simulink model "hmi_view_manager_02"  (Simulink 7.0)
settings: Solver=ode45  StartTime=0.0  StopTime=inf  RelTol=1e-3
settings Model: Creator=emanoj1  LastModifiedBy=ARAJASE2

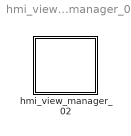
== system hmi_view_manager_02 ==
  hmi_view_manager_02 : Stateflow chart

== stateflow chart hmi_view_manager_02 ==
  settings: executeAtInitialization=1
  state VM_LOGIC_ST [parallel]
    /*
    ** Maintains the request from HMI logic
    */
    settings: executionOrder=1
    state VM_LOGIC_ACTIVE_ST
      entry:
      l_logic_active_state_id = p_logic_req_state_id;
      l_logic_active_anim_id = p_logic_req_anim_id;
      exit:
      l_logic_active_state_id = LSH_ALL_VM_LOGIC_STATES;
      l_logic_active_anim_id = ANIM_MAX_ID;
      VM_LOGIC_ACTIVE_ST -> (junction 29) [order 1] : LSH_LOGIC_ADD_EV
          | [p_logic_req_state_id < LSH_ALL_VM_LOGIC_STATES]
      (junction 29) -> (junction 30) [order 1] : /* New state is replacing current state */
          | [l_logic_active_state_id != p_logic_req_state_id]
      (junction 61) -> (junction 34)
      (junction 29) -> (junction 32) [order 2] : /* requested state is same as active state */
      (junction 30) -> (junction 33) [order 1] : [(p_logic_req_state_id == l_gfx_active_state_id) &&...
          | (!in(VM_GFX_CLOSE_ANIM_ST))]
          | {l_gfx_deactivate_flag = FALSE;}
      (junction 31) -> (junction 34) [order 2] : /*
          | ** active state is not being presented yet by graphics
          | ** so no deactivations required
          | */
      (junction 32) -> (junction 33) [order 2] : /* req state prev anim actively running */
      (junction 34) -> (junction 33)
      (junction 33) -> VM_LOGIC_ACTIVE_ST : {
          |    l_logic_active_state_id = p_logic_req_state_id;
          |    l_logic_active_anim_id = p_logic_req_anim_id;
          | }
      (junction 32) -> (junction 64) [order 1] : [(l_gfx_active_anim_id == ANIM_MAX_ID) ]
          | {
          | $#ifdef LSH_IGNORE_ANIM_REQUEST_DURING_ACTIVE_ANIM$
          |    l_logic_active_anim_id = ANIM_MAX_ID;
          | $#else$
          |    l_logic_active_anim_id = p_logic_req_anim_id;
          | $#endif$
          | }
      (junction 30) -> (junction 31) [order 2]
      (junction 31) -> (junction 60) [order 1] : /*
          | ** active state is being presented by graphics so
          | ** need to deactivate it
          | */
          | [l_logic_active_state_id == l_gfx_active_state_id]
          | {l_gfx_deactivate_flag = TRUE;
          |  l_gfx_deactivate_anim = ANIM_MAX_ID;}
      (junction 60) -> (junction 61)
      (junction 64) -> VM_LOGIC_ACTIVE_ST [order 2]
      (junction 64) -> (junction 62) [order 1] : [l_logic_active_anim_id ==ANIM_ABORT_ID]
      (junction 62) -> VM_LOGIC_ACTIVE_ST : {
          |  l_logic_active_anim_id = ANIM_MAX_ID;
          | }
    state VM_LOGIC_INACTIVE_ST
      (junction 73) -> VM_LOGIC_INACTIVE_ST [order 1] : [ (p_logic_req_anim_id==ANIM_ABORT_ID)]
          | {l_gfx_deactivate_anim = p_logic_req_anim_id;}
      VM_LOGIC_INACTIVE_ST -> (junction 68) [order 1] : LSH_LOGIC_REMOVE_EV
          | [(p_logic_req_state_id == l_gfx_active_state_id) ]
      (junction 68) -> (junction 69) [order 1] : [! in(VM_GFX_CLOSE_ANIM_ST)]
      (junction 69) -> VM_LOGIC_INACTIVE_ST : {l_gfx_deactivate_anim = p_logic_req_anim_id;}
      (junction 68) -> (junction 73) [order 2]
      (junction 73) -> (junction 74) [order 2]
      (junction 74) -> VM_LOGIC_INACTIVE_ST : /* Do Nothing*/
          | /* QAC 8.1.2 Fix*/
    (default) -> VM_LOGIC_INACTIVE_ST
    VM_LOGIC_INACTIVE_ST -> (junction 25) [order 1] : LSH_LOGIC_ADD_EV
        | [p_logic_req_state_id < LSH_ALL_VM_LOGIC_STATES]
    (junction 25) -> VM_LOGIC_ACTIVE_ST
    (junction 27) -> VM_LOGIC_INACTIVE_ST [order 1] : [p_logic_req_state_id == l_gfx_active_state_id]
        | {l_gfx_deactivate_flag = TRUE;
        |  l_gfx_deactivate_anim = p_logic_req_anim_id;}
    VM_LOGIC_ACTIVE_ST -> (junction 27) [order 1] : LSH_LOGIC_REMOVE_EV
        | [p_logic_req_state_id == l_logic_active_state_id]
    (junction 27) -> (junction 28) [order 2]
    (junction 28) -> VM_LOGIC_INACTIVE_ST
  state VM_PRESENTATION_ST [parallel]
    /*
    ** Maintains the graphics state
    */
    settings: executionOrder=2
    state VM_GFX_ACTIVE_ST
      entry:
      l_gfx_prev_focus = 0;
      l_gfx_deactivate_flag = FALSE;
      state VM_GFX_NORMAL_RUN_ST
        state VM_GFX_ACTIVE_PRESENT_ST
          entry:
          l_logic_active_anim_id = ANIM_MAX_ID; /*Added during Abort anim implementation */
          hmi_vm_focus(l_gfx_active_state_id, ...
          (LSH_GOT_FOCUS_STATUS|LSH_ANIM_COMPLETE_STATUS));
          hmi_lsh_run_presentation(l_gfx_active_state_id,l_gfx_presentation_state);
          l_gfx_presentation_state = LSH_REFRESH_STATUS;
          /*Added during Abort anim implementation */
          l_gfx_active_anim_id = ANIM_MAX_ID;
          VM_GFX_ACTIVE_PRESENT_ST -> (junction 65) : /* call refresh every alternate cycles */
              | LSH_GFX_TICK_EV
              | {hmi_lsh_run_presentation(l_gfx_active_state_id, LSH_REFRESH_STATUS);}
          (junction 65) -> VM_GFX_ACTIVE_PRESENT_ST [order 1] : [l_logic_active_anim_id==ANIM_ABORT_ID]
              | {l_logic_active_anim_id = ANIM_MAX_ID;}
          (junction 66) -> VM_GFX_ACTIVE_PRESENT_ST
          (junction 65) -> (junction 66) [order 2]
        state VM_GFX_ACTIVE_ANIMATION_ST
          entry:
          hmi_vm_focus(l_gfx_active_state_id,(LSH_GOT_FOCUS_STATUS|LSH_ANIM_STARTED_STATUS));
          on LSH_GFX_FORCE_PRESENTATION_EV:
          hmi_lsh_run_presentation(l_gfx_active_state_id,l_gfx_presentation_state);
          l_gfx_presentation_state = LSH_REFRESH_STATUS;
        (junction 48) -> (junction 41) [order 1] : [l_logic_active_anim_id < ANIM_MAX_ID]
        (default) -> (junction 48)
        (junction 41) -> (junction 40) : {
            |    hmi_lsh_stop_animation(l_gfx_active_state_id, l_gfx_active_anim_id);
            |    l_gfx_active_anim_id     = l_logic_active_anim_id;
            |    l_logic_active_anim_id  = ANIM_MAX_ID;
            | }
        (junction 40) -> VM_GFX_ACTIVE_ANIMATION_ST [order 1] : /*
            | ** !!!!! This transition needs to be avaluated first always
            | ** So if for any chance if you rearrange the states
            | ** please make sure the order is maintained
            | */
            | [hmi_lsh_start_animation(l_gfx_active_state_id, l_gfx_active_anim_id) != FALSE]
        (junction 63) -> (junction 41)
        VM_GFX_NORMAL_RUN_ST -> (junction 63) : LSH_GFX_TICK_EV
            | [l_logic_active_anim_id < ANIM_MAX_ID]
            | /* if logic active state is different, it will exit
            | in parent state  */
        (junction 47) -> VM_GFX_ACTIVE_PRESENT_ST : [!in(VM_GFX_ACTIVE_PRESENT_ST)]
        VM_GFX_ACTIVE_ANIMATION_ST -> (junction 63) [order 1] : LSH_ANIM_COMPLETE_EV
        (junction 40) -> (junction 47) [order 2]
        (junction 48) -> VM_GFX_ACTIVE_PRESENT_ST [order 2]
        (junction 42) -> (junction 47) : LSH_GFX_TICK_EV
            | [(l_logic_active_anim_id==ANIM_ABORT_ID)&&...
            |         (l_gfx_active_state_id==l_logic_active_state_id)]
            | {
            | hmi_lsh_stop_animation(l_gfx_active_state_id, l_gfx_active_anim_id);
            | l_logic_active_anim_id=ANIM_MAX_ID;
            | }
        VM_GFX_ACTIVE_ANIMATION_ST -> (junction 42) [order 2]
      state VM_GFX_STARTUP_ANIM_ST
        entry:
        hmi_vm_focus(l_gfx_active_state_id, (LSH_GOT_FOCUS_STATUS|LSH_ANIM_STARTED_STATUS));
        on LSH_GFX_FORCE_PRESENTATION_EV:
        hmi_lsh_run_presentation(l_gfx_active_state_id,l_gfx_presentation_state);
        l_gfx_presentation_state = LSH_REFRESH_STATUS;
      note: When entering for the first time see if we need to run a startup anim
          | While doing startup anim, if there is a request to run presentaion do it.
          | Once the startup anim is complete, enter normal  mode and do
          | presentation
          | In normal mode if the animation is requested perform that
      (default) -> (junction 43)
      (junction 35) -> VM_GFX_NORMAL_RUN_ST [order 1] : /* no animations */
          | [hmi_lsh_start_animation(l_gfx_active_state_id, l_gfx_active_anim_id)==FALSE]
      (junction 35) -> (junction 36) [order 2]
      VM_GFX_STARTUP_ANIM_ST -> VM_GFX_NORMAL_RUN_ST [order 2] : LSH_ANIM_COMPLETE_EV
      (junction 36) -> VM_GFX_STARTUP_ANIM_ST
      VM_GFX_ACTIVE_ST -> (junction 43) [order 1] : LSH_GFX_TICK_EV
          | [(l_gfx_active_state_id != l_logic_active_state_id)]
          | {
          |    l_gfx_prev_focus = 0;
          |    hmi_lsh_run_presentation(l_gfx_active_state_id, ...
          |                                        LSH_DEACTIVATED_STATUS);
          |    hmi_vm_focus(l_gfx_active_state_id, ...
          |                                (LSH_LOST_FOCUS_STATUS|...
          |                                 LSH_DEACTIVATED_STATUS|...
          |                                 LSH_ANIM_COMPLETE_STATUS));
          |    hmi_lsh_freeze_button_events_ext(LSH_GET_STATE_ID(l_gfx_active_state_id), ...
          |                                                                     LSH_GET_CLIENT_ID(l_gfx_active_state_id));
          | }
          | /*
          | Force a reentry if the logic state is different than
          | the current graphics state
          | This path is never expected to execute
          | */
      (junction 43) -> (junction 35) : {
          |    hmi_lsh_stop_animation(l_gfx_active_state_id, l_gfx_active_anim_id);
          |    l_gfx_active_state_id       = l_logic_active_state_id;
          |    l_gfx_active_anim_id       = l_logic_active_anim_id;
          |    l_logic_active_anim_id    = ANIM_MAX_ID;
          |    l_gfx_presentation_state = LSH_ACTIVATED_STATUS;
          | }
      VM_GFX_STARTUP_ANIM_ST -> VM_GFX_NORMAL_RUN_ST [order 1] : LSH_GFX_TICK_EV
          | [(l_logic_active_anim_id==ANIM_ABORT_ID)&&...
          |         (l_gfx_active_state_id==l_logic_active_state_id)]
          | {
          | hmi_lsh_stop_animation(l_gfx_active_state_id, l_gfx_active_anim_id);
          | l_logic_active_anim_id=ANIM_MAX_ID;
          | }
    state VM_GFX_INACTIVE_ST
      entry:
      l_gfx_active_state_id     = LSH_ALL_VM_LOGIC_STATES;
      l_gfx_active_anim_id     = ANIM_MAX_ID;
    state VM_GFX_CLOSE_ANIM_ST
      entry:
      l_gfx_active_anim_id = l_gfx_deactivate_anim;
      l_gfx_deactivate_anim = ANIM_MAX_ID;
    (default) -> VM_GFX_INACTIVE_ST
    VM_GFX_INACTIVE_ST -> VM_GFX_ACTIVE_ST : /* Check if we have got a new logic state */
        | LSH_GFX_TICK_EV
        | [l_logic_active_state_id < LSH_ALL_VM_LOGIC_STATES]
    VM_GFX_ACTIVE_ST -> (junction 37) [order 1] : /*
        | ** If the logic state has gone inactive or if the deactivation flag is set
        | ** then perform a deactivation. Perform the animation if requested
        | */
        | LSH_GFX_TICK_EV||...
        | LSH_GFX_CHECK_DEACTIVATION_EV||...
        | LSH_ANIM_COMPLETE_EV
        | [(l_logic_active_state_id == LSH_ALL_VM_LOGIC_STATES) || ...
        |  (l_gfx_deactivate_flag != FALSE)]
        | {
        |     hmi_lsh_stop_animation(l_gfx_active_state_id, l_gfx_active_anim_id);
        | }
    (junction 37) -> VM_GFX_CLOSE_ANIM_ST [order 1] : [hmi_lsh_start_animation(l_gfx_active_state_id, l_gfx_deactivate_anim) != FALSE]
    (junction 37) -> (junction 72) [order 2] : /* Animation not started */
    (junction 38) -> (junction 44) [order 2]
    VM_GFX_CLOSE_ANIM_ST -> (junction 39) [order 2] : /* animation completed and no state active */
        | LSH_ANIM_COMPLETE_EV
    (junction 39) -> (junction 72)
    (junction 44) -> VM_GFX_INACTIVE_ST [order 2]
    (junction 44) -> VM_GFX_ACTIVE_ST [order 1] : /* if we come here via l_gfx_deactivate_flag != FALSE path
        |    then check to see if there is an active state beccause
        |   focus handler can add/remove states */
        | [l_logic_active_state_id < LSH_ALL_VM_LOGIC_STATES]
    (junction 67) -> (junction 39)
    VM_GFX_CLOSE_ANIM_ST -> (junction 67) [order 1] : LSH_GFX_TICK_EV
        | [l_gfx_deactivate_anim==ANIM_ABORT_ID]
        | {
        |      hmi_lsh_stop_animation(l_gfx_active_state_id, l_gfx_active_anim_id);
        |     l_gfx_deactivate_anim=ANIM_MAX_ID;
        | }
    (junction 38) -> (junction 71) [order 1] : [(l_gfx_active_state_id != l_logic_active_state_id)]
    (junction 71) -> (junction 70) : {
        | hmi_lsh_freeze_button_events_ext(LSH_GET_STATE_ID(l_gfx_active_state_id), ...
        |                                                  LSH_GET_CLIENT_ID(l_gfx_active_state_id));
        | }
    (junction 70) -> (junction 44)
    (junction 72) -> (junction 38) : {
        | hmi_lsh_run_presentation(l_gfx_active_state_id,LSH_DEACTIVATED_STATUS);
        |    hmi_vm_focus(l_gfx_active_state_id, ...
        |                              (LSH_LOST_FOCUS_STATUS|...
        |                               LSH_DEACTIVATED_STATUS|...
        |                               LSH_ANIM_COMPLETE_STATUS));
        | }
  state hmi_vm_focus(p_state_id, p_focus) [function]
    (junction 54) -> (junction 26) : {
        |    hmi_lsh_focus_handler(p_state_id, p_focus);
        |    l_gfx_prev_focus = p_focus;
        | }
    (default) -> (junction 54)
  state hmi_vm_tick [function]
    (default) -> (junction 45) : {
        |    send(LSH_GFX_TICK_EV, VM_PRESENTATION_ST);
        |    send(LSH_GFX_TICK_EV, VM_PERIODIC_FOCUS_MONITOR_ST);
        | }
  state hmi_vm_check_deactivation [function]
    (default) -> (junction 50) : {
        |    send(LSH_GFX_CHECK_DEACTIVATION_EV, VM_PRESENTATION_ST);
        | }
  state hmi_vm_animation_completed [function]
    (default) -> (junction 53) : {
        |    send(LSH_ANIM_COMPLETE_EV, VM_PRESENTATION_ST);
        | }
  state hmi_vm_force_presentation [function]
    (default) -> (junction 46) : {
        |    send(LSH_GFX_FORCE_PRESENTATION_EV, VM_PRESENTATION_ST);
        | }
  state VM_PERIODIC_FOCUS_MONITOR_ST [parallel]
    settings: executionOrder=3
    note: This state will periodically invoke the focus handler to make sure that if a higher priority state got deactivated
        | then if this is the active state, appropriately set the got focus notification. Because the deactivated high
        | priority state will not initiate a got focus notification for next low priority state. It is this peridic check that
        | detects and generates the notification in such case
    VM_PERIODIC_FOCUS_MONITOR_ST -> (junction 49) : LSH_GFX_TICK_EV
        | [!in(VM_GFX_INACTIVE_ST)]
    (junction 49) -> VM_PERIODIC_FOCUS_MONITOR_ST : [hmi_lsh_get_focus_status(LSH_GET_STATE_ID(l_gfx_active_state_id)) == LSH_FOCUS_STATUS_INACTIVE]
        | {hmi_vm_focus(l_gfx_active_state_id, l_gfx_prev_focus);}
  state hmi_vm_add_state(p_state_id, p_anim_id) [function]
    (default) -> (junction 51) : {
        |    p_logic_req_state_id = p_state_id;
        |    p_logic_req_anim_id = p_anim_id;
        |    send(LSH_LOGIC_ADD_EV, VM_LOGIC_ST);
        | }
  state hmi_vm_remove_state(p_state_id, p_anim_id) [function]
    (default) -> (junction 52) : {
        |    p_logic_req_state_id = p_state_id;
        |    p_logic_req_anim_id = p_anim_id;
        |    send(LSH_LOGIC_REMOVE_EV, VM_LOGIC_ST);
        | }
  state r_anim_active = hmi_vm_animation_active_status [function]
    (default) -> (junction 55)
    (junction 55) -> (junction 56) [order 1] : [in(VM_GFX_STARTUP_ANIM_ST) ||...
        |  (in(VM_GFX_ACTIVE_ANIMATION_ST)) ||...
        |  (in(VM_GFX_CLOSE_ANIM_ST))]
        | { r_anim_active=TRUE; }
    (junction 55) -> (junction 57) [order 2]
    (junction 57) -> (junction 58) : {r_anim_active=FALSE;}
    (junction 56) -> (junction 58)
    (junction 58) -> (junction 59)
  data: p_state_id function_input uint16; p_focus function_input uint8; p_state_id function_input uint16; p_anim_id function_input uint8; p_state_id function_input uint16; p_anim_id function_input uint8; r_anim_active function_output boolean; p_logic_req_state_id local uint16 =65535; p_logic_req_anim_id local uint8 =255; l_logic_active_state_id local uint16 =65535; l_logic_active_anim_id local uint8 =255; l_gfx_active_state_id local uint16 =65535; l_gfx_active_anim_id local uint8 =255; l_gfx_deactivate_flag local uint8 =0; l_gfx_deactivate_anim local uint8 =255; l_priority local uint8 =255; l_gfx_prev_focus local uint8 =0; l_gfx_presentation_state local uint8 =0
  data p_logic_req_state_id settings: description=Temporarily holds the requested logic state
  data p_logic_req_anim_id settings: description=Temporarily holds the requested animation ID
  data l_logic_active_state_id settings: description=Holds the state ID for the logic state added by application.
  data l_logic_active_anim_id settings: description=Holds the animation ID for the logic state added by application
  data l_gfx_active_state_id settings: description=This variable holds the active state id for which the graphics is built or going to get built
  data l_gfx_active_anim_id settings: description=This variable holds the active graphics state's animation id for which the graphics is built or going to get built
  data l_gfx_deactivate_flag settings: description=If this flag is true indicates that the currently active graphics state (l_gfx_active_state_id) needs to be deactivated
  data l_gfx_deactivate_anim settings: description=This variable holds the active graphics state's deactivation animation id for which the graphics is built or going to g
  data l_priority settings: description=Holds the current logic states priority
  data l_gfx_prev_focus settings: description=Indicates the last focus status sent to active state
  data l_gfx_presentation_state settings: description=|
      | Indicates the presentation state (activate, refresh, deactivate) to be passed on to the l_gfx_active_state_id's presentation handler
      | This is introduced to fic the issue that the activate getting called multiple times due to forced presentation during animation
  events: LSH_GFX_TICK_EV local EITHER_EDGE_EVENT; LSH_ANIM_COMPLETE_EV local EITHER_EDGE_EVENT; LSH_LOGIC_ADD_EV local EITHER_EDGE_EVENT; LSH_LOGIC_REMOVE_EV local EITHER_EDGE_EVENT; LSH_GFX_FORCE_PRESENTATION_EV local EITHER_EDGE_EVENT; LSH_GFX_CHECK_DEACTIVATION_EV local EITHER_EDGE_EVENT
